simulink model "UDP_connection"  (R2020a)
settings: Solver=VariableStepAuto  StartTime=0.0  StopTime=10.0  RelTol=1e-3
undefined symbols (not defined in the file): f
libraries: instrumentlib x2
settings Model: EnablePacing=on  Creator=JClae  LastModifiedBy=JClae

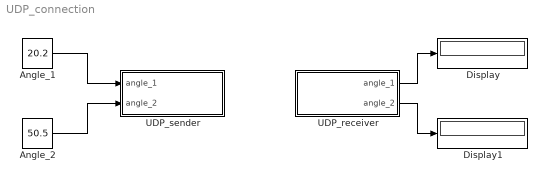
== system UDP_connection ==
  Angle_1 : Constant  Value=20.2  OutMin=0  OutMax=360  OutDataTypeStr=double
  Angle_2 : Constant  Value=50.5  OutMin=0  OutMax=360  OutDataTypeStr=double
  Display : Display
  Display1 : Display
  UDP_receiver : Subsystem
  UDP_sender : Subsystem
  wires:
  Angle_1/1 -> UDP_sender/1(angle_1)
  Angle_2/1 -> UDP_sender/2(angle_2)
  UDP_receiver/1(angle_1) -> Display/1
  UDP_receiver/2(angle_2) -> Display1/1

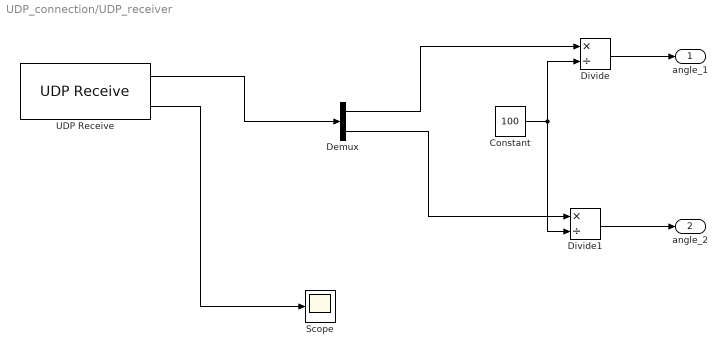
== system UDP_connection/UDP_receiver ==
  Constant : Constant  Value=100
  Demux : Demux  Outputs=2
  Divide : Product  Inputs=*/
  Divide1 : Product  Inputs=*/
  Scope : Scope
  UDP Receive : instrumentlib/UDP Receive  Host=localhost  Port=9090  LocalPort=8888  EnablePortSharing=off  GetLatestData=off  DataSize="[2  1]"  DataType=int16  ASCIIFormatting=%f,  Terminator=LF  ByteOrder=BigEndian  EnableBlockingMode=off  Timeout=10  SampleTime=0.1  LocalAddress=localhost
  angle_1 : Outport
  angle_2 : Outport  Port=2
  wires:
  Demux/2 -> Divide1/1
  Divide1/1 -> angle_2/1
  UDP Receive/1 -> Demux/1
  UDP Receive/2 -> Scope/1
  Divide/1 -> angle_1/1
  Demux/1 -> Divide/1
  Constant/1 -> Divide1/2, Divide/2

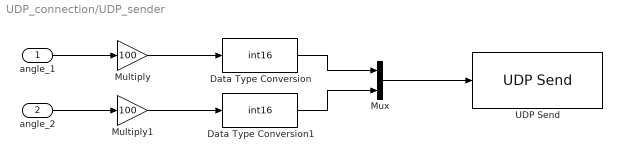
== system UDP_connection/UDP_sender ==
  angle_1 : Inport
  angle_2 : Inport  Port=2
  Data Type Conversion : DataTypeConversion  OutDataTypeStr=int16
  Data Type Conversion1 : DataTypeConversion  OutDataTypeStr=int16
  Multiply : Gain  Gain=100
  Multiply1 : Gain  Gain=100
  Mux : Mux  Inputs=2
  UDP Send : instrumentlib/UDP Send  Host=localhost  Port=8888  LocalPort=-1  EnablePortSharing=off  ByteOrder=BigEndian  OutputDatagramPacketSize=512  EnableBlockingMode=off  LocalAddress=0.0.0.0
  wires:
  Multiply1/1 -> Data Type Conversion1/1
  Mux/1 -> UDP Send/1
  Data Type Conversion1/1 -> Mux/2
  Data Type Conversion/1 -> Mux/1
  angle_2/1 -> Multiply1/1
  Multiply/1 -> Data Type Conversion/1
  angle_1/1 -> Multiply/1
